simulink model "system5"  (R2018b)
settings: Solver=VariableStepAuto  StartTime=0.0  StopTime=1  MaxStep=.001  RelTol=1e-3
libraries: cstblocks x8
settings Model: Creator=Abraham Pérez  LastModifiedBy=Abraham Pérez

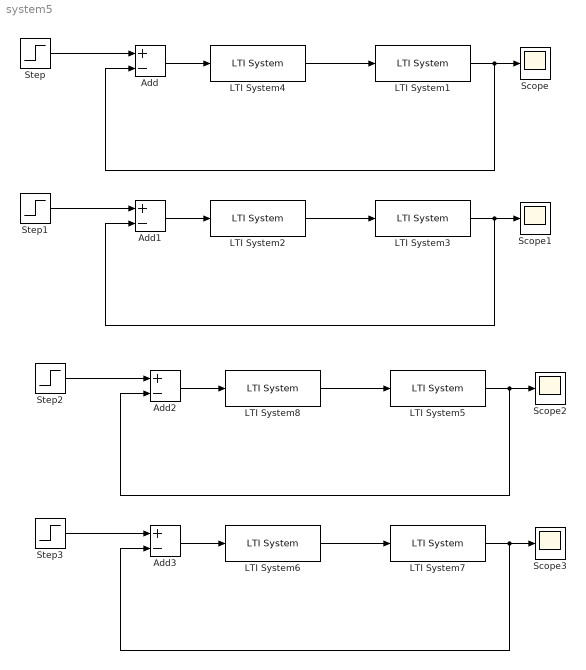
== system system5 ==
  Add{,1..3} (4 alike) : Sum  Inputs=+-
  LTI System1 : cstblocks/LTI System  sys=G5_H1  IC=[]
  LTI System2 : cstblocks/LTI System  sys=C5_H1Lag  IC=[]
  LTI System3 : cstblocks/LTI System  sys=G5_H1  IC=[]
  LTI System4 : cstblocks/LTI System  sys=C5_H1Lead  IC=[]
  LTI System5 : cstblocks/LTI System  sys=G5_H2  IC=[]
  LTI System6 : cstblocks/LTI System  sys=C5_H2Lag  IC=[]
  LTI System7 : cstblocks/LTI System  sys=G5_H2  IC=[]
  LTI System8 : cstblocks/LTI System  sys=C5_H2Lead  IC=[]
  Scope{,1..3} (4 alike) : Scope
  Step : Step  Time=0  After=17  SampleTime=0
  Step1 : Step  Time=0  After=9  SampleTime=0
  Step2 : Step  Time=0  After=17  SampleTime=0
  Step3 : Step  Time=0  After=9  SampleTime=0
  wires:
  Add/1 -> LTI System4/1
  LTI System4/1 -> LTI System1/1
  LTI System3/1 -> Add1/2, Scope1/1
  Step1/1 -> Add1/1
  LTI System2/1 -> LTI System3/1
  LTI System1/1 -> Add/2, Scope/1
  Step/1 -> Add/1
  Add1/1 -> LTI System2/1
  Step2/1 -> Add2/1
  Add3/1 -> LTI System6/1
  Step3/1 -> Add3/1
  LTI System5/1 -> Add2/2, Scope2/1
  LTI System6/1 -> LTI System7/1
  LTI System7/1 -> Add3/2, Scope3/1
  Add2/1 -> LTI System8/1
  LTI System8/1 -> LTI System5/1
